simulink model "lookupTableDynamic_TestGen33"  (R2017b)
settings: Solver=FixedStepDiscrete  StartTime=0.0  StopTime=10.0  RelTol=1e-3
libraries: simulink x1
settings Model: Creator=ktrinh  LastModifiedBy=ktrinh
settings DebuggingCC: ParameterOverflowMsg=none

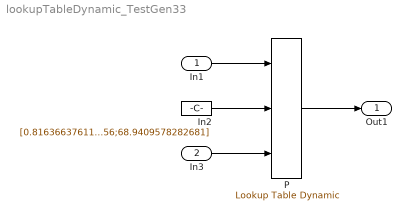
== system lookupTableDynamic_TestGen33 ==
  In1 : Inport  OutMin=-1.1836  OutMax=70.941  OutDataTypeStr=double  PortDimensions=1
  In3 : Inport  Port=2  PortDimensions=5
  In2 : Constant  Value=[0.81636637611798;24.0342735111896;27.4704734918631;67.1916015602356;68.9409578282681]  OutDataTypeStr=double
  P : simulink/Lookup Tables/Lookup Table Dynamic  LookUpMeth=Use Input Above  OutDataType=fixdt('uint16')  OutScaling=[]  OutputDataTypeScalingMode=Specify via dialog  OutDataTypeStr=uint16  RndMeth=Simplest  DoSatur=on
      settings: SourceProductName=Simulink
  Out1 : Outport
  wires:
  In1/1 -> P/1
  In2/1 -> P/2
  In3/1 -> P/3
  P/1 -> Out1/1
